simulink model "H_Bridge_Direct_PWM"  (Simulink 7.5)
settings: Solver=ode23  StartTime=0.0  StopTime=10.0  RelTol=1e-3
libraries: powerlib x8, powerlib_extras x3, simulink x2
settings Model: Creator=lm  LastModifiedBy=lm

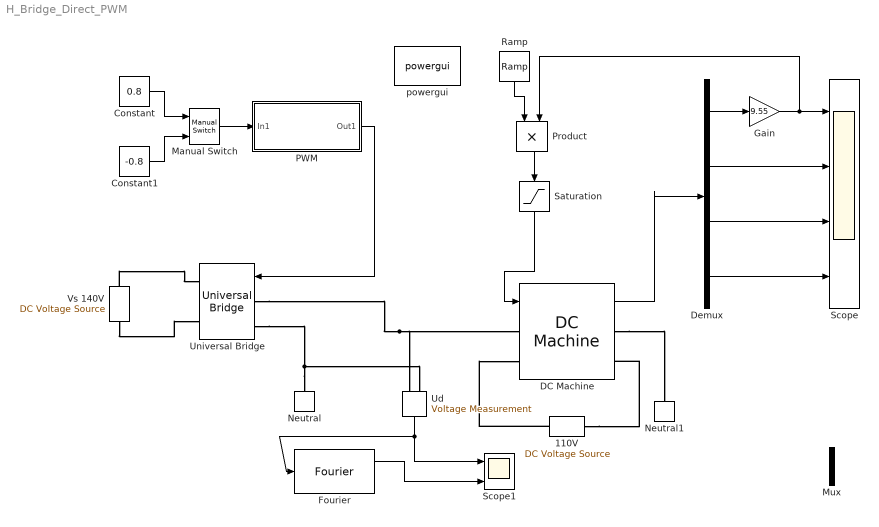
== system H_Bridge_Direct_PWM ==
  110V : powerlib/Electrical Sources/DC Voltage Source  DialogController=POWERSYS.PowerSysDialog  SystemSampleTime=-1  Amplitude=110  Measurements=None
  Constant : Constant  Value=0.8  OutDataType=fixdt(1, 16)  OutScaling=2^0
  Constant1 : Constant  Value=-0.8  OutDataType=fixdt(1, 16)  OutScaling=2^0
  DC Machine : powerlib/Machines/DC Machine  DialogController=POWERSYS.PowerSysDialog  SystemSampleTime=-1  PresetModel=No  MechanicalLoad=Torque TL  FieldType=Wound  ShowDetailedParameters=on  RLa="[ 3.4  0.0604]"  RLf="[ 220  0]"  Laf=0.797  MachineConstant=Torque constant (N.m/A)  Ke=1.8  Kt=1.8  J=0.014  Bm=0  Tf=0  w0=1  Ifinit=1  TsPowergui=0  TsBlock=-1
      settings: AttributesFormatString=\n
  Demux : Demux
  Fourier : powerlib_extras/Measurements/Fourier  DialogController=POWERSYS.PowerSysDialog  SystemSampleTime=-1  f1=1080  n=0
  Gain : Gain  Gain=9.55  ParameterDataType=fixdt(1, 16)  ParameterScaling=2^0  OutDataType=fixdt(1, 16)  OutScaling=2^0
  Manual Switch : simulink/Signal Routing/Manual Switch  SystemSampleTime=-1  sw=1  action=0  varsize=off
  Mux : Mux  Inputs=2
  Neutral : powerlib/Elements/Neutral  DialogController=POWERSYS.PowerSysDialog  PhysicalDomain=powersysdomain  SubClassName=unknown  LeftPortType=p1  RightPortType=p1  LConnTagsString=a  NodeNumber=99
  Neutral1 : powerlib/Elements/Neutral  DialogController=POWERSYS.PowerSysDialog  PhysicalDomain=powersysdomain  SubClassName=unknown  LeftPortType=p1  RightPortType=p1  LConnTagsString=a  NodeNumber=99
  PWM : Subsystem
  Product : Product  OutDataType=fixdt(1, 16)  OutScaling=2^0  RndMeth=Zero
  Ramp : simulink/Sources/Ramp  SystemSampleTime=-1  slope=1000  start=0  X0=0
  Saturation : Saturate  UpperLimit=1.15  LowerLimit=-1.15  OutDataType=fixdt(1, 16)  OutScaling=2^0
  Scope : Scope  NumInputPorts=4
      settings: YMin=0.25~-1~0.5~-0.4  YMax=3.5~1~0.5~0.4
  Scope1 : Scope  NumInputPorts=2
      settings: YMin=-150~53.75  YMax=150~59.5
  Ud : powerlib/Measurements/Voltage Measurement  DialogController=POWERSYS.PowerSysDialog  SystemSampleTime=-1  PhasorSimulation=off  OutputType=Complex  PSBequivalent=0
  Universal Bridge : powerlib/Power Electronics/Universal Bridge  DialogController=POWERSYS.PowerSysDialog  SystemSampleTime=-1  Arms=2  SnubberResistance=1e5  SnubberCapacitance=inf  Device=MOSFET / Diodes  Ron=1e-3  Lon=0  ForwardVoltages="[  0  0  ]"  ForwardVoltage=0  GTOparameters=[ 10e-6 , 20e-6 ]  IGBTparameters=[ 1e-6 , 2e-6 ]  Measurements=None  Measurements_2=None  converterType=Rectifier
  Vs 140V : powerlib/Electrical Sources/DC Voltage Source  DialogController=POWERSYS.PowerSysDialog  SystemSampleTime=-1  Amplitude=140  Measurements=None
  powergui : powerlib/powergui  Priority=1  SystemSampleTime=-1  SimulationMode=Discrete  SampleTime=50e-6  frequency=60  SPID=off  DisableSnubberDevices=off  DisableRonSwitches=off  DisableVfSwitches=off  SwTol=0  Interpol=off  frequencyindice=0  echomessages=off  HookPort=off  DisplayEquations=off  FunctionMessages=off  EnableUseOfTLC=off  x0status=blocks  RestoreLinks=warning  ResistiveCurrentMeasurement=off  Ylog=off  Xlog=on  ShowGrid=off  save=off  variable=ZData  ZoomFFT=off  StartTime=0.0  cycles=1  DisplayStyle=1  FreqAxis=off  MaxFrequency=1000  frequencyindicesteady=1  display=off  methode=off
  wires:
  Constant/1 -> Manual Switch/1
  Constant1/1 -> Manual Switch/2
  Manual Switch/1 -> PWM/1(In1)
  PWM/1(Out1) -> Universal Bridge/1
  DC Machine/1 -> Demux/1
  Demux/1 -> Gain/1
  Gain/1 -> Scope/1, Product/2
  Demux/2 -> Scope/2
  Demux/3 -> Scope/3
  Demux/4 -> Scope/4
  Ud/1 -> Scope1/1, Fourier/1
  Fourier/1 -> Scope1/2
  Saturation/1 -> DC Machine/1
  Product/1 -> Saturation/1
  Ramp/1 -> Product/1
  connections:
  Vs 140V/LConn1 -- Universal Bridge/RConn2
  Vs 140V/RConn1 -- Universal Bridge/RConn1
  110V/RConn1 -- DC Machine/LConn2
  110V/LConn1 -- DC Machine/RConn2
  Neutral/LConn1 -- Universal Bridge/LConn2 -- Ud/LConn2
  Universal Bridge/LConn1 -- DC Machine/LConn1 -- Ud/LConn1
  DC Machine/RConn1 -- Neutral1/LConn1

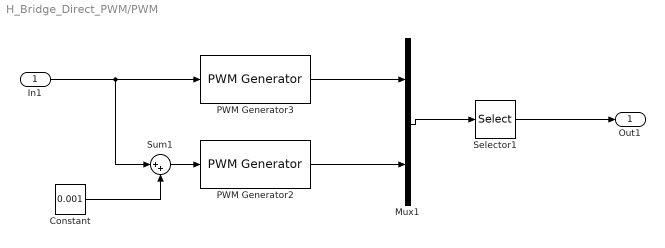
== system H_Bridge_Direct_PWM/PWM ==
  In1 : Inport  OutDataType=fixdt(1, 16)  OutScaling=2^0
  Constant : Constant  Value=0.001  OutDataType=fixdt(1, 16)  OutScaling=2^0
  Mux1 : Mux  Inputs=2
  PWM Generator2 : powerlib_extras/Control  Blocks/PWM Generator  DialogController=POWERSYS.PowerSysDialog  SystemSampleTime=-1  GeneratorMode="1-arm  bridge (2 pulses)"  Fc=1080  Internal=off  mIndex=0.4  Freq=60  Phase=0
  PWM Generator3 : powerlib_extras/Control  Blocks/PWM Generator  DialogController=POWERSYS.PowerSysDialog  SystemSampleTime=-1  GeneratorMode="1-arm  bridge (2 pulses)"  Fc=1080  Internal=off  mIndex=0.4  Freq=60  Phase=0
  Selector1 : Selector  InputPortWidth=4  IndexOptions=Index vector (dialog)  Indices=[1 2 4 3]  OutputSizes=1
  Sum1 : Sum  Inputs=|++  OutDataType=fixdt(1, 16)  OutScaling=2^0
  Out1 : Outport  OutDataType=fixdt(1, 16)  OutScaling=2^0
  wires:
  Selector1/1 -> Out1/1
  Mux1/1 -> Selector1/1
  PWM Generator2/1 -> Mux1/2
  PWM Generator3/1 -> Mux1/1
  Sum1/1 -> PWM Generator2/1
  Constant/1 -> Sum1/2
  In1/1 -> PWM Generator3/1, Sum1/1
